simulink model "Punto3c"  (R2017b)
settings: Solver=VariableStepAuto  StartTime=0.0  StopTime=10  RelTol=1e-3
libraries: simulink x1
settings Model: Creator=Agustin  LastModifiedBy=Agustin

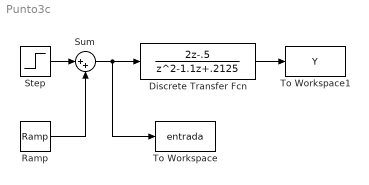
== system Punto3c ==
  Discrete Transfer Fcn : DiscreteTransferFcn  Numerator=[0 2 -.5]  Denominator=[1 -1.1 .2125]  SampleTime=1
  Ramp : simulink/Sources/Ramp  slope=1  start=2  X0=0
  Step : Step  SampleTime=0
  Sum : Sum  Inputs=|++
  To Workspace : ToWorkspace  VariableName=entrada  SaveFormat=Timeseries  SampleTime=-1
  To Workspace1 : ToWorkspace  VariableName=Y  SaveFormat=Timeseries  SampleTime=-1
  wires:
  Discrete Transfer Fcn/1 -> To Workspace1/1
  Ramp/1 -> Sum/2
  Step/1 -> Sum/1
  Sum/1 -> To Workspace/1, Discrete Transfer Fcn/1
